simulink model "Scenario_17_v2"  (R2020b)
settings: Solver=ode1  StartTime=0.0  StopTime=10  FixedStep=Ts  MaxStep=Ts  MinStep=Ts/50  RelTol=1e-3
values from neighbouring files (symbols this model uses):
  c0 = c0_zeb    (= 6.57988e-09)    [Scenario_17_parameters_v2.m]    (also in Scenario_1_parameters_v2.m; Scenario_2_parameters_v2.m; Scenario_3_parameters_v2.m)
  c1 = c1_zeb    (= 9.15905e-09)    [Scenario_17_parameters_v2.m]    (also in Scenario_1_parameters_v2.m; Scenario_2_parameters_v2.m; Scenario_3_parameters_v2.m)
  fg = 50    [Scenario_17_parameters_v2.m]    (also in Scenario_1_parameters_v2.m; Scenario_2_parameters_v2.m; Scenario_3_parameters_v2.m)
  G11gen = 0.50    (= 0.5)    [Scenario_17_parameters_v2.m]
  G1gen = 0.4692    [Scenario_17_parameters_v2.m]    (also in Scenario_1_parameters_v2.m = 0.1; Scenario_2_parameters_v2.m = 0.298581; Scenario_3_parameters_v2.m = 0.65)
  G5gen = 0.75    [Scenario_17_parameters_v2.m]    (also in Scenario_1_parameters_v2.m = 0.8; Scenario_2_parameters_v2.m = 0.8; Scenario_3_parameters_v2.m = 0.705)
  G6gen = 0.90    (= 0.9)    [Scenario_17_parameters_v2.m]    (also in Scenario_1_parameters_v2.m; Scenario_2_parameters_v2.m = 0.81797; Scenario_3_parameters_v2.m = 0.45)
  G7gen = 0.20    (= 0.2)    [Scenario_17_parameters_v2.m]    (also in Scenario_1_parameters_v2.m = 0.5227; Scenario_2_parameters_v2.m = 0.5098; Scenario_3_parameters_v2.m = 0.4)
  G8gen = 0.58    [Scenario_17_parameters_v2.m]    (also in Scenario_3_parameters_v2.m = 0.65)
  G9gen = 0.8833    [Scenario_17_parameters_v2.m]    (also in Scenario_3_parameters_v2.m = 0.9)
  Iovc = 1.2    [Scenario_17_parameters_v2.m]    (also in Scenario_1_parameters_v2.m; Scenario_2_parameters_v2.m; Scenario_3_parameters_v2.m)
  l0 = l0_zeb    (= 0.00368)    [Scenario_17_parameters_v2.m]    (also in Scenario_1_parameters_v2.m; Scenario_2_parameters_v2.m; Scenario_3_parameters_v2.m)
  l1 = l1_zeb    (= 0.00128)    [Scenario_17_parameters_v2.m]    (also in Scenario_1_parameters_v2.m; Scenario_2_parameters_v2.m; Scenario_3_parameters_v2.m)
  L11dem = 0.02    [Scenario_17_parameters_v2.m]
  L12dem = 0.01    [Scenario_17_parameters_v2.m]    (also in Scenario_3_parameters_v2.m = 0.02)
  L1dem = 0.25    [Scenario_17_parameters_v2.m]    (also in Scenario_3_parameters_v2.m = 0.1)
  L3dem = 0.30    (= 0.3)    [Scenario_17_parameters_v2.m]    (also in Scenario_1_parameters_v2.m = 0.1; Scenario_2_parameters_v2.m = 0.1; Scenario_3_parameters_v2.m = 0.2)
  L5dem = 0.25    [Scenario_17_parameters_v2.m]    (also in Scenario_1_parameters_v2.m = 0.35; Scenario_2_parameters_v2.m = 0.35; Scenario_3_parameters_v2.m = 0.1)
  L9dem = 0.15    [Scenario_17_parameters_v2.m]    (also in Scenario_3_parameters_v2.m = 0.1)
  Pr = Sr*PF    (= 1600500000)    [Scenario_17_parameters_v2.m]    (also in Scenario_1_parameters_v2.m = 1472500000; Scenario_2_parameters_v2.m = 1805000000; Scenario_3_parameters_v2.m = 12740000000)
  Qr = sqrt(Sr^2 - Pr^2)    [Scenario_17_parameters_v2.m]    (also in Scenario_1_parameters_v2.m; Scenario_2_parameters_v2.m; Scenario_3_parameters_v2.m)
  r0 = r0_zeb    (= 0.39362)    [Scenario_17_parameters_v2.m]    (also in Scenario_1_parameters_v2.m; Scenario_2_parameters_v2.m; Scenario_3_parameters_v2.m)
  r1 = r1_zeb    (= 0.06862)    [Scenario_17_parameters_v2.m]    (also in Scenario_1_parameters_v2.m; Scenario_2_parameters_v2.m; Scenario_3_parameters_v2.m)
  Rtpu = Xtpu/40    (= 0.0025)    [Scenario_17_parameters_v2.m]    (also in Scenario_1_parameters_v2.m = 0.00375; Scenario_2_parameters_v2.m = 0.00375; Scenario_3_parameters_v2.m)
  S11non = 50e6    (= 50000000)    [Scenario_17_parameters_v2.m]
  S1non = 700e6    (= 700000000)    [Scenario_17_parameters_v2.m]    (also in Scenario_1_parameters_v2.m = 400000000; Scenario_2_parameters_v2.m = 400000000; Scenario_3_parameters_v2.m = 1000000000)
  S5non = 400e6    (= 400000000)    [Scenario_17_parameters_v2.m]    (also in Scenario_1_parameters_v2.m = 500000000; Scenario_2_parameters_v2.m = 500000000; Scenario_3_parameters_v2.m = 2000000000)
  S6non = 150e6    (= 150000000)    [Scenario_17_parameters_v2.m]    (also in Scenario_1_parameters_v2.m = 400000000; Scenario_2_parameters_v2.m = 400000000; Scenario_3_parameters_v2.m = 3000000000)
  S7non = 1500e6    (= 1500000000)    [Scenario_17_parameters_v2.m]    (also in Scenario_1_parameters_v2.m = 200000000; Scenario_2_parameters_v2.m = 200000000; Scenario_3_parameters_v2.m = 4000000000)
  S8non = 600e6    (= 600000000)    [Scenario_17_parameters_v2.m]    (also in Scenario_3_parameters_v2.m = 2000000000)
  S9non = 200e6    (= 200000000)    [Scenario_17_parameters_v2.m]    (also in Scenario_3_parameters_v2.m = 1500000000)
  tonvsc = 0    [Scenario_17_parameters_v2.m]    (also in Scenario_1_parameters_v2.m; Scenario_2_parameters_v2.m; Scenario_3_parameters_v2.m = 0.0001)
  Ts = 50e-6    (= 5e-05)    [Scenario_17_parameters_v2.m]    (also in Scenario_1_parameters_v2.m = 0.0002; Scenario_2_parameters_v2.m = 2e-05; Scenario_3_parameters_v2.m = 0.0001)
  Vhv = 220e3    (= 220000)    [Scenario_17_parameters_v2.m]    (also in Scenario_1_parameters_v2.m; Scenario_2_parameters_v2.m; Scenario_3_parameters_v2.m)
  Vmv = 22e3    (= 22000)    [Scenario_17_parameters_v2.m]    (also in Scenario_1_parameters_v2.m; Scenario_2_parameters_v2.m; Scenario_3_parameters_v2.m)
  w_pll = 2*pi*80    (= 502.654824574)    [Scenario_17_parameters_v2.m]    (also in Scenario_1_parameters_v2.m; Scenario_2_parameters_v2.m; Scenario_3_parameters_v2.m)
  wc1 = wsw1/10    (= 848.230016469)    [Scenario_17_parameters_v2.m]    (also in Scenario_1_parameters_v2.m; Scenario_2_parameters_v2.m; Scenario_3_parameters_v2.m)
  wdc1 = wc1/10    (= 84.8230016469)    [Scenario_17_parameters_v2.m]    (also in Scenario_1_parameters_v2.m; Scenario_2_parameters_v2.m; Scenario_3_parameters_v2.m)
  wpq1 = wc1/10    (= 84.8230016469)    [Scenario_17_parameters_v2.m]    (also in Scenario_1_parameters_v2.m; Scenario_2_parameters_v2.m; Scenario_3_parameters_v2.m)
  wsw1 = ksw1*2*pi*fg    (= 8482.30016469)    [Scenario_17_parameters_v2.m]    (also in Scenario_1_parameters_v2.m; Scenario_2_parameters_v2.m; Scenario_3_parameters_v2.m)
  Xtpu = 0.10    (= 0.1)    [Scenario_17_parameters_v2.m]    (also in Scenario_1_parameters_v2.m = 0.15; Scenario_2_parameters_v2.m = 0.15; Scenario_3_parameters_v2.m)
undefined symbols (not defined in the file or in its folder): D11, Delta, Newton, Raphson
libraries: powerlib x349, simulink_extras x215, powerlib_meascontrol x165, pid_lib x81, simulink x48, eeTransforms x42, spsFirstOrderFilterLib x28, eePwmGeneratorTwoLevel x7
(part 4 of 31)

== system Scenario_17_v2/HVDC 1 ==
  note: Converter controlling DC voltage
  note: DC Link dynamics
  note: avoid division by zero
  note: avoid division by zero
  Bus Selector1 : BusSelector  OutputSignals=Pabc,Qabc,f
  Bus Selector2 : BusSelector  OutputSignals=Pabc,Qabc,f
  Constant : Constant  Value=-S7non*G7gen
  Constant1 : Constant  Value=0
  Constant2 : Constant  Value=100e6
  DC-link : Subsystem  mask{C1=3100e-6/2, C2=3100e-6/2, R=4, L=100e-3, Vdc0=2*Vhv*sqrt(2)/sqrt(3), Pdc0=S7non*G7gen}
      mask prompts: C1 "Terminal 1 capacitance (F)"; C2 "Termina 2 capacitance (F)"; R "Link series resistance (Ohm)"; L "Link series inductance (H)"; Vdc0 "Link Initial voltage (V)"; Pdc0 "Initial power flowing from 1 to 2"
      mask init:
      | idc0 = Pdc0/Vdc0;
      | v2dc0 = Vdc0; % Initial voltage of terminal 2
      | v1dc0 = Vdc0 + idc0*R; % Initial voltage of terminal 1
      mask Display:
      | disp('back-to-back\n')
      | disp('\nDC link')
  Divide : Product  Inputs=*/
  Divide1 : Product  Inputs=*/
  Gain1 : Gain  Gain=-1
  Gain2 : Gain  Gain=-1
  Saturation : Saturate  UpperLimit=5*Vhv  LowerLimit=0.01*Vhv
  Saturation1 : Saturate  UpperLimit=5*Vhv  LowerLimit=0.01*Vhv
  Unit Delay : UnitDelay  SampleTime=-1  HasFrameUpgradeWarning=on
  Unit Delay1 : UnitDelay  SampleTime=-1  HasFrameUpgradeWarning=on
  VSC1 : Subsystem  mask{vscmod=EMT Average, fg=fg, Vhv=Vhv, Vmv=Vhv, Pconv=S7non, Rtpu=Rtpu, Xtpu=Xtpu, qmode=Active power, dmode=Reactive power, wsw=wsw1, wn_pll=w_pll, wc=wc1, wpq=wpq1, wdc=wdc1, koc=Iovc, Cdc=3100e-6, tfilt=1*(1/wsw1), negseq_en=off, fdroop_en=off, Vacdroop_en=off, LVRT_en=off, Kfdroop=0.05, fdroop_per=10, Kvdroop=0.1, Vacdroop_per=10, Vlvrt0=0.9, Vlvrt_min=0.5, Qmax_lvrt=0.9, V0pu=1, theta0=0, P0=-S7non*G7gen, Q0=0}
      mask prompts: vscmod "VSC Model"; fg "AC grid frequency (Hz)"; Vhv "Grid-side voltage (V)(LL-rms)"; Vmv "Converter-side voltage (V)(LL-rms)"; Pconv "Converter nominal power (VA)"; Rtpu "Resistance seen by the converter (p.u)"; Xtpu "Reactance seen by the converter (p.u)"; qmode "q-axis control mode"; dmode "d-axis control mode"; wsw "Switching frequency (rad/s)"; wn_pll "PLL filter natural frequency"; wc "Current-control bandwidth (rad/s)"; wpq "PQ control bandwidth (rad/s)"; wdc "DC Voltage control bandwidth(rad/s)"; koc "Overcurrent factor (p.u)"; Cdc "DC-side total capacitance (F)"; tfilt "Vabc filter time constant (s)"; negseq_en "Enable negative sequence control"; fdroop_en "Enable frequency droop"; Vacdroop_en "Enable AC voltage droop"; LVRT_en "Enable LVRT"; Kfdroop "Frequency droop (p.u)"; fdroop_per "Percentage of converter power to contribute with droop (%)"; Kvdroop "Voltage droop (p.u)"; Vacdroop_per "Percentage of converter power to contribute with droop (%)"; Vlvrt0 "initial voltage (p.u)"; Vlvrt_min "minimum voltage (p.u)"; Qmax_lvrt "max power injected at min voltage (p.u)"; V0pu "Initial terminal voltage magnitude (pu)"; theta0 "Initial terminal voltage angle (deg)"; P0 "Initial active power (W)"; Q0 "Initial reactive power (VAr)"
      mask init: same as Scenario_17_v2/G11new/VSC v2
      mask TypeOptions vscmod: EMT Switching | EMT Average | Phasor Quasi-EMT | Phasor I-1st | Phasor I-ref | Phasor PQ-1st
      mask Callback vscmod:
      | % Control parameter visiblity
      | 
      | % Get the value of the Enable Bias checkbox
      | % unchecked = 'off'
      | % checked = 'on'
      | 
      | maskObj = Simulink.Mask.get(gcb);
      | 
      | wn_pll = 'on';
      | wsw = 'on';
      | DC_en = 'off';
      | 
      | vscmod = get_param(gcb,'vscmod');
      |     if strcmp(vscmod,'EMT Switching')
      |       wn_pll = 'on';
      |       wsw = 'on';
      |       tfilt = 'on';
      |     elseif strcmp(vscmod,'EMT Average')
      |         wn_pll = 'on';
      |         wsw = 'off';
      |         tfilt = 'off';
      |     elseif strcmp(vscmod,'Phasor Quasi-EMT')
      |         wn_pll = 'off';
      |         wsw = 'off';
      |         tfilt = 'off';
      |     elseif strcmp(vscmod,'Phasor I-1st')
      |         wn_pll = 'off';
      |         wsw = 'off';
      |         tfilt = 'off';
      |     elseif strcmp(vscmod,'Phasor I-ref')
      |         wn_pll = 'off';
      |         wsw = 'off';
      |         tfilt = 'off';
      |     elseif strcmp(vscmod,'Phasor PQ-1st')
      |         wn_pll = 'off';
      |         wsw = 'off';
      |         tfilt = 'off';
      |     end
      | 
      | fdroop_en = get_param(gcb,'fdroop_en');
      | Vacdroop_en = get_param(gcb,'Vacdroop_en');
      | LVRT_en = get_param(gcb,'LVRT_en');
      | negseq_en = get_param(gcb,'negseq_en');
      | qmode_str = get_param(gcb,'qmode');
      | 
      | 
      | if strcmp(qmode_str,'DC voltage')
      |     DC_en = 'on';
      | else
      |     DC_en = 'off';
      | end
      | 
      | % Set the 'MaskVisibilities' property for each parameters
      |     set_param(gcb,'MaskVisibilities',{'on','on','on','on','on','on','on','on','on',wsw,wn_pll,'on','on','on','on',DC_en,tfilt,'on','on','on','on',fdroop_en,fdroop_en,Vacdroop_en,Vacdroop_en,'on','on','on','on','on','on','on'});
      | 
      | % Make LVRT area visible when it is enabled
      | if strcmp(LVRT_en,'on')
      |   maskObj.getDialogControl('Container_LVRT').Visible = 'on';
      | else
      |     maskObj.getDialogControl('Container_LVRT').Visible = 'off';
      | end
      | 
      | % Note that the value of the bias is not handled here.
      | % See the Initialization tab
      mask TypeOptions qmode: Active power | DC voltage
      mask Callback qmode:
      | % Control parameter visiblity
      | 
      | % Get the value of the Enable Bias checkbox
      | % unchecked = 'off'
      | % checked = 'on'
      | 
      | maskObj = Simulink.Mask.get(gcb);
      | 
      | wn_pll = 'on';
      | wsw = 'on';
      | DC_en = 'off';
      | 
      | vscmod = get_param(gcb,'vscmod');
      |     if strcmp(vscmod,'EMT Switching')
      |       wn_pll = 'on';
      |       wsw = 'on';
      |       tfilt = 'on';
      |     elseif strcmp(vscmod,'EMT Average')
      |         wn_pll = 'on';
      |         wsw = 'off';
      |         tfilt = 'off';
      |     elseif strcmp(vscmod,'Phasor Quasi-EMT')
      |         wn_pll = 'off';
      |         wsw = 'off';
      |         tfilt = 'off';
      |     elseif strcmp(vscmod,'Phasor I-1st')
      |         wn_pll = 'off';
      |         wsw = 'off';
      |         tfilt = 'off';
      |     elseif strcmp(vscmod,'Phasor I-ref')
      |         wn_pll = 'off';
      |         wsw = 'off';
      |         tfilt = 'off';
      |     elseif strcmp(vscmod,'Phasor PQ-1st')
      |         wn_pll = 'off';
      |         wsw = 'off';
      |         tfilt = 'off';
      |     end
      | 
      | fdroop_en = get_param(gcb,'fdroop_en');
      | Vacdroop_en = get_param(gcb,'Vacdroop_en');
      | LVRT_en = get_param(gcb,'LVRT_en');
      | negseq_en = get_param(gcb,'negseq_en');
      | qmode_str = get_param(gcb,'qmode');
      | 
      | 
      | if strcmp(qmode_str,'DC voltage')
      |     DC_en = 'on';
      | else
      |     DC_en = 'off';
      | end
      | 
      | % Set the 'MaskVisibilities' property for each parameters
      |     set_param(gcb,'MaskVisibilities',{'on','on','on','on','on','on','on','on','on',wsw,wn_pll,'on','on','on','on',DC_en,tfilt,'on','on','on','on',fdroop_en,fdroop_en,Vacdroop_en,Vacdroop_en,'on','on','on','on','on','on','on'});
      | 
      | % Make LVRT area visible when it is enabled
      | if strcmp(LVRT_en,'on')
      |   maskObj.getDialogControl('Container_LVRT').Visible = 'on';
      | else
      |     maskObj.getDialogControl('Container_LVRT').Visible = 'off';
      | end
      | 
      | % Note that the value of the bias is not handled here.
      | % See the Initialization tab
      mask TypeOptions dmode: Reactive power | AC voltage
      mask Callback fdroop_en:
      | % Control parameter visiblity
      | 
      | % Get the value of the Enable Bias checkbox
      | % unchecked = 'off'
      | % checked = 'on'
      | 
      | maskObj = Simulink.Mask.get(gcb);
      | 
      | wn_pll = 'on';
      | wsw = 'on';
      | DC_en = 'off';
      | 
      | vscmod = get_param(gcb,'vscmod');
      |     if strcmp(vscmod,'EMT Switching')
      |       wn_pll = 'on';
      |       wsw = 'on';
      |       tfilt = 'on';
      |     elseif strcmp(vscmod,'EMT Average')
      |         wn_pll = 'on';
      |         wsw = 'off';
      |         tfilt = 'off';
      |     elseif strcmp(vscmod,'Phasor Quasi-EMT')
      |         wn_pll = 'off';
      |         wsw = 'off';
      |         tfilt = 'off';
      |     elseif strcmp(vscmod,'Phasor I-1st')
      |         wn_pll = 'off';
      |         wsw = 'off';
      |         tfilt = 'off';
      |     elseif strcmp(vscmod,'Phasor I-ref')
      |         wn_pll = 'off';
      |         wsw = 'off';
      |         tfilt = 'off';
      |     elseif strcmp(vscmod,'Phasor PQ-1st')
      |         wn_pll = 'off';
      |         wsw = 'off';
      |         tfilt = 'off';
      |     end
      | 
      | fdroop_en = get_param(gcb,'fdroop_en');
      | Vacdroop_en = get_param(gcb,'Vacdroop_en');
      | LVRT_en = get_param(gcb,'LVRT_en');
      | negseq_en = get_param(gcb,'negseq_en');
      | qmode_str = get_param(gcb,'qmode');
      | 
      | 
      | if strcmp(qmode_str,'DC voltage')
      |     DC_en = 'on';
      | else
      |     DC_en = 'off';
      | end
      | 
      | % Set the 'MaskVisibilities' property for each parameters
      |     set_param(gcb,'MaskVisibilities',{'on','on','on','on','on','on','on','on','on',wsw,wn_pll,'on','on','on','on',DC_en,tfilt,'on','on','on','on',fdroop_en,fdroop_en,Vacdroop_en,Vacdroop_en,'on','on','on','on','on','on','on'});
      | 
      | % Make LVRT area visible when it is enabled
      | if strcmp(LVRT_en,'on')
      |   maskObj.getDialogControl('Container_LVRT').Visible = 'on';
      | else
      |     maskObj.getDialogControl('Container_LVRT').Visible = 'off';
      | end
      | 
      | % Note that the value of the bias is not handled here.
      | % See the Initialization tab
      mask Callback Vacdroop_en:
      | % Control parameter visiblity
      | 
      | % Get the value of the Enable Bias checkbox
      | % unchecked = 'off'
      | % checked = 'on'
      | 
      | maskObj = Simulink.Mask.get(gcb);
      | 
      | wn_pll = 'on';
      | wsw = 'on';
      | DC_en = 'off';
      | 
      | vscmod = get_param(gcb,'vscmod');
      |     if strcmp(vscmod,'EMT Switching')
      |       wn_pll = 'on';
      |       wsw = 'on';
      |       tfilt = 'on';
      |     elseif strcmp(vscmod,'EMT Average')
      |         wn_pll = 'on';
      |         wsw = 'off';
      |         tfilt = 'off';
      |     elseif strcmp(vscmod,'Phasor Quasi-EMT')
      |         wn_pll = 'off';
      |         wsw = 'off';
      |         tfilt = 'off';
      |     elseif strcmp(vscmod,'Phasor I-1st')
      |         wn_pll = 'off';
      |         wsw = 'off';
      |         tfilt = 'off';
      |     elseif strcmp(vscmod,'Phasor I-ref')
      |         wn_pll = 'off';
      |         wsw = 'off';
      |         tfilt = 'off';
      |     elseif strcmp(vscmod,'Phasor PQ-1st')
      |         wn_pll = 'off';
      |         wsw = 'off';
      |         tfilt = 'off';
      |     end
      | 
      | fdroop_en = get_param(gcb,'fdroop_en');
      | Vacdroop_en = get_param(gcb,'Vacdroop_en');
      | LVRT_en = get_param(gcb,'LVRT_en');
      | negseq_en = get_param(gcb,'negseq_en');
      | qmode_str = get_param(gcb,'qmode');
      | 
      | 
      | if strcmp(qmode_str,'DC voltage')
      |     DC_en = 'on';
      | else
      |     DC_en = 'off';
      | end
      | 
      | % Set the 'MaskVisibilities' property for each parameters
      |     set_param(gcb,'MaskVisibilities',{'on','on','on','on','on','on','on','on','on',wsw,wn_pll,'on','on','on','on',DC_en,tfilt,'on','on','on','on',fdroop_en,fdroop_en,Vacdroop_en,Vacdroop_en,'on','on','on','on','on','on','on'});
      | 
      | % Make LVRT area visible when it is enabled
      | if strcmp(LVRT_en,'on')
      |   maskObj.getDialogControl('Container_LVRT').Visible = 'on';
      | else
      |     maskObj.getDialogControl('Container_LVRT').Visible = 'off';
      | end
      | 
      | % Note that the value of the bias is not handled here.
      | % See the Initialization tab
      mask Callback LVRT_en:
      | % Control parameter visiblity
      | 
      | % Get the value of the Enable Bias checkbox
      | % unchecked = 'off'
      | % checked = 'on'
      | 
      | maskObj = Simulink.Mask.get(gcb);
      | 
      | wn_pll = 'on';
      | wsw = 'on';
      | DC_en = 'off';
      | 
      | vscmod = get_param(gcb,'vscmod');
      |     if strcmp(vscmod,'EMT Switching')
      |       wn_pll = 'on';
      |       wsw = 'on';
      |       tfilt = 'on';
      |     elseif strcmp(vscmod,'EMT Average')
      |         wn_pll = 'on';
      |         wsw = 'off';
      |         tfilt = 'off';
      |     elseif strcmp(vscmod,'Phasor Quasi-EMT')
      |         wn_pll = 'off';
      |         wsw = 'off';
      |         tfilt = 'off';
      |     elseif strcmp(vscmod,'Phasor I-1st')
      |         wn_pll = 'off';
      |         wsw = 'off';
      |         tfilt = 'off';
      |     elseif strcmp(vscmod,'Phasor I-ref')
      |         wn_pll = 'off';
      |         wsw = 'off';
      |         tfilt = 'off';
      |     elseif strcmp(vscmod,'Phasor PQ-1st')
      |         wn_pll = 'off';
      |         wsw = 'off';
      |         tfilt = 'off';
      |     end
      | 
      | fdroop_en = get_param(gcb,'fdroop_en');
      | Vacdroop_en = get_param(gcb,'Vacdroop_en');
      | LVRT_en = get_param(gcb,'LVRT_en');
      | negseq_en = get_param(gcb,'negseq_en');
      | qmode_str = get_param(gcb,'qmode');
      | 
      | 
      | if strcmp(qmode_str,'DC voltage')
      |     DC_en = 'on';
      | else
      |     DC_en = 'off';
      | end
      | 
      | % Set the 'MaskVisibilities' property for each parameters
      |     set_param(gcb,'MaskVisibilities',{'on','on','on','on','on','on','on','on','on',wsw,wn_pll,'on','on','on','on',DC_en,tfilt,'on','on','on','on',fdroop_en,fdroop_en,Vacdroop_en,Vacdroop_en,'on','on','on','on','on','on','on'});
      | 
      | % Make LVRT area visible when it is enabled
      | if strcmp(LVRT_en,'on')
      |   maskObj.getDialogControl('Container_LVRT').Visible = 'on';
      | else
      |     maskObj.getDialogControl('Container_LVRT').Visible = 'off';
      | end
      | 
      | % Note that the value of the bias is not handled here.
      | % See the Initialization tab
      mask DialogControl DescTextVar Prompt: -------------------------------------Three-phase VSC model---------------------------------------
      mask DialogControl Tab1 Prompt: Electrical parameters
      mask DialogControl Tab2 Prompt: Control parameters
      mask DialogControl Tab3 Prompt: Other parameters
      mask DialogControl Container_LVRT Prompt: LVRT
      mask DialogControl Tab4 Prompt: Power flow
      mask Display:
      | choice = get_param(gcb,'vscmod');
      | if strcmp(choice,'Phasor Quasi-EMT')
      |     disp('VSC\n\n')
      |     disp('\n\nPhasor\n\n')
      |     disp('\n\nQuasi-EMT')
      | elseif strcmp(choice,'EMT Average')
      |     disp('VSC\n')
      |     disp('\nEMT AVG')
      | elseif strcmp(choice,'EMT Switching')
      |     disp('VSC\n')
      |     disp('\nEMT SW')
      | elseif strcmp(choice,'Phasor I-1st')
      |     disp('VSC\n\n')
      |     disp('\n\nPhasor\n\n')
      |     disp('\n\nI 1st')
      | elseif strcmp(choice,'Phasor I-ref')
      |     disp('VSC\n\n')
      |     disp('\n\nPhasor\n\n')
      |     disp('\n\nI ref')
      | elseif strcmp(choice,'Phasor PQ-1st')
      |     disp('VSC\n\n')
      |     disp('\n\nPhasor\n\n')
      |     disp('\n\nPQ 1st')
      | end
  VSC2 : Subsystem  mask{vscmod=EMT Average, fg=fg, Vhv=Vhv, Vmv=Vhv, Pconv=S7non, Rtpu=Rtpu, Xtpu=Xtpu, qmode=DC voltage, dmode=Reactive power, wsw=wsw1, wn_pll=w_pll, wc=wc1, wpq=wpq1, wdc=wdc1, koc=Iovc, Cdc=3100e-6, tfilt=1*(1/wsw1), negseq_en=off, fdroop_en=off, Vacdroop_en=off, LVRT_en=off, Kfdroop=0.05, fdroop_per=10, Kvdroop=0.1, Vacdroop_per=10, Vlvrt0=0.9, Vlvrt_min=0.5, Qmax_lvrt=0.9, V0pu=1.0433, theta0=-29.85, P0=S7non*G7gen, Q0=100e6}
      mask prompts: vscmod "VSC Model"; fg "AC grid frequency (Hz)"; Vhv "Grid-side voltage (V)(LL-rms)"; Vmv "Converter-side voltage (V)(LL-rms)"; Pconv "Converter nominal power (VA)"; Rtpu "Resistance seen by the converter (p.u)"; Xtpu "Reactance seen by the converter (p.u)"; qmode "q-axis control mode"; dmode "d-axis control mode"; wsw "Switching frequency (rad/s)"; wn_pll "PLL filter natural frequency"; wc "Current-control bandwidth (rad/s)"; wpq "PQ control bandwidth (rad/s)"; wdc "DC Voltage control bandwidth(rad/s)"; koc "Overcurrent factor (p.u)"; Cdc "DC-side total capacitance (F)"; tfilt "Vabc filter time constant (s)"; negseq_en "Enable negative sequence control"; fdroop_en "Enable frequency droop"; Vacdroop_en "Enable AC voltage droop"; LVRT_en "Enable LVRT"; Kfdroop "Frequency droop (p.u)"; fdroop_per "Percentage of converter power to contribute with droop (%)"; Kvdroop "Voltage droop (p.u)"; Vacdroop_per "Percentage of converter power to contribute with droop (%)"; Vlvrt0 "initial voltage (p.u)"; Vlvrt_min "minimum voltage (p.u)"; Qmax_lvrt "max power injected at min voltage (p.u)"; V0pu "Initial terminal voltage magnitude (pu)"; theta0 "Initial terminal voltage angle (deg)"; P0 "Initial active power (W)"; Q0 "Initial reactive power (VAr)"
      mask init: same as Scenario_17_v2/G11new/VSC v2
      mask TypeOptions vscmod: EMT Switching | EMT Average | Phasor Quasi-EMT | Phasor I-1st | Phasor I-ref | Phasor PQ-1st
      mask Callback vscmod:
      | % Control parameter visiblity
      | 
      | % Get the value of the Enable Bias checkbox
      | % unchecked = 'off'
      | % checked = 'on'
      | 
      | maskObj = Simulink.Mask.get(gcb);
      | 
      | wn_pll = 'on';
      | wsw = 'on';
      | DC_en = 'off';
      | 
      | vscmod = get_param(gcb,'vscmod');
      |     if strcmp(vscmod,'EMT Switching')
      |       wn_pll = 'on';
      |       wsw = 'on';
      |       tfilt = 'on';
      |     elseif strcmp(vscmod,'EMT Average')
      |         wn_pll = 'on';
      |         wsw = 'off';
      |         tfilt = 'off';
      |     elseif strcmp(vscmod,'Phasor Quasi-EMT')
      |         wn_pll = 'off';
      |         wsw = 'off';
      |         tfilt = 'off';
      |     elseif strcmp(vscmod,'Phasor I-1st')
      |         wn_pll = 'off';
      |         wsw = 'off';
      |         tfilt = 'off';
      |     elseif strcmp(vscmod,'Phasor I-ref')
      |         wn_pll = 'off';
      |         wsw = 'off';
      |         tfilt = 'off';
      |     elseif strcmp(vscmod,'Phasor PQ-1st')
      |         wn_pll = 'off';
      |         wsw = 'off';
      |         tfilt = 'off';
      |     end
      | 
      | fdroop_en = get_param(gcb,'fdroop_en');
      | Vacdroop_en = get_param(gcb,'Vacdroop_en');
      | LVRT_en = get_param(gcb,'LVRT_en');
      | negseq_en = get_param(gcb,'negseq_en');
      | qmode_str = get_param(gcb,'qmode');
      | 
      | 
      | if strcmp(qmode_str,'DC voltage')
      |     DC_en = 'on';
      | else
      |     DC_en = 'off';
      | end
      | 
      | % Set the 'MaskVisibilities' property for each parameters
      |     set_param(gcb,'MaskVisibilities',{'on','on','on','on','on','on','on','on','on',wsw,wn_pll,'on','on','on','on',DC_en,tfilt,'on','on','on','on',fdroop_en,fdroop_en,Vacdroop_en,Vacdroop_en,'on','on','on','on','on','on','on'});
      | 
      | % Make LVRT area visible when it is enabled
      | if strcmp(LVRT_en,'on')
      |   maskObj.getDialogControl('Container_LVRT').Visible = 'on';
      | else
      |     maskObj.getDialogControl('Container_LVRT').Visible = 'off';
      | end
      | 
      | % Note that the value of the bias is not handled here.
      | % See the Initialization tab
      mask TypeOptions qmode: Active power | DC voltage
      mask Callback qmode:
      | % Control parameter visiblity
      | 
      | % Get the value of the Enable Bias checkbox
      | % unchecked = 'off'
      | % checked = 'on'
      | 
      | maskObj = Simulink.Mask.get(gcb);
      | 
      | wn_pll = 'on';
      | wsw = 'on';
      | DC_en = 'off';
      | 
      | vscmod = get_param(gcb,'vscmod');
      |     if strcmp(vscmod,'EMT Switching')
      |       wn_pll = 'on';
      |       wsw = 'on';
      |       tfilt = 'on';
      |     elseif strcmp(vscmod,'EMT Average')
      |         wn_pll = 'on';
      |         wsw = 'off';
      |         tfilt = 'off';
      |     elseif strcmp(vscmod,'Phasor Quasi-EMT')
      |         wn_pll = 'off';
      |         wsw = 'off';
      |         tfilt = 'off';
      |     elseif strcmp(vscmod,'Phasor I-1st')
      |         wn_pll = 'off';
      |         wsw = 'off';
      |         tfilt = 'off';
      |     elseif strcmp(vscmod,'Phasor I-ref')
      |         wn_pll = 'off';
      |         wsw = 'off';
      |         tfilt = 'off';
      |     elseif strcmp(vscmod,'Phasor PQ-1st')
      |         wn_pll = 'off';
      |         wsw = 'off';
      |         tfilt = 'off';
      |     end
      | 
      | fdroop_en = get_param(gcb,'fdroop_en');
      | Vacdroop_en = get_param(gcb,'Vacdroop_en');
      | LVRT_en = get_param(gcb,'LVRT_en');
      | negseq_en = get_param(gcb,'negseq_en');
      | qmode_str = get_param(gcb,'qmode');
      | 
      | 
      | if strcmp(qmode_str,'DC voltage')
      |     DC_en = 'on';
      | else
      |     DC_en = 'off';
      | end
      | 
      | % Set the 'MaskVisibilities' property for each parameters
      |     set_param(gcb,'MaskVisibilities',{'on','on','on','on','on','on','on','on','on',wsw,wn_pll,'on','on','on','on',DC_en,tfilt,'on','on','on','on',fdroop_en,fdroop_en,Vacdroop_en,Vacdroop_en,'on','on','on','on','on','on','on'});
      | 
      | % Make LVRT area visible when it is enabled
      | if strcmp(LVRT_en,'on')
      |   maskObj.getDialogControl('Container_LVRT').Visible = 'on';
      | else
      |     maskObj.getDialogControl('Container_LVRT').Visible = 'off';
      | end
      | 
      | % Note that the value of the bias is not handled here.
      | % See the Initialization tab
      mask TypeOptions dmode: Reactive power | AC voltage
      mask Callback fdroop_en:
      | % Control parameter visiblity
      | 
      | % Get the value of the Enable Bias checkbox
      | % unchecked = 'off'
      | % checked = 'on'
      | 
      | maskObj = Simulink.Mask.get(gcb);
      | 
      | wn_pll = 'on';
      | wsw = 'on';
      | DC_en = 'off';
      | 
      | vscmod = get_param(gcb,'vscmod');
      |     if strcmp(vscmod,'EMT Switching')
      |       wn_pll = 'on';
      |       wsw = 'on';
      |       tfilt = 'on';
      |     elseif strcmp(vscmod,'EMT Average')
      |         wn_pll = 'on';
      |         wsw = 'off';
      |         tfilt = 'off';
      |     elseif strcmp(vscmod,'Phasor Quasi-EMT')
      |         wn_pll = 'off';
      |         wsw = 'off';
      |         tfilt = 'off';
      |     elseif strcmp(vscmod,'Phasor I-1st')
      |         wn_pll = 'off';
      |         wsw = 'off';
      |         tfilt = 'off';
      |     elseif strcmp(vscmod,'Phasor I-ref')
      |         wn_pll = 'off';
      |         wsw = 'off';
      |         tfilt = 'off';
      |     elseif strcmp(vscmod,'Phasor PQ-1st')
      |         wn_pll = 'off';
      |         wsw = 'off';
      |         tfilt = 'off';
      |     end
      | 
      | fdroop_en = get_param(gcb,'fdroop_en');
      | Vacdroop_en = get_param(gcb,'Vacdroop_en');
      | LVRT_en = get_param(gcb,'LVRT_en');
      | negseq_en = get_param(gcb,'negseq_en');
      | qmode_str = get_param(gcb,'qmode');
      | 
      | 
      | if strcmp(qmode_str,'DC voltage')
      |     DC_en = 'on';
      | else
      |     DC_en = 'off';
      | end
      | 
      | % Set the 'MaskVisibilities' property for each parameters
      |     set_param(gcb,'MaskVisibilities',{'on','on','on','on','on','on','on','on','on',wsw,wn_pll,'on','on','on','on',DC_en,tfilt,'on','on','on','on',fdroop_en,fdroop_en,Vacdroop_en,Vacdroop_en,'on','on','on','on','on','on','on'});
      | 
      | % Make LVRT area visible when it is enabled
      | if strcmp(LVRT_en,'on')
      |   maskObj.getDialogControl('Container_LVRT').Visible = 'on';
      | else
      |     maskObj.getDialogControl('Container_LVRT').Visible = 'off';
      | end
      | 
      | % Note that the value of the bias is not handled here.
      | % See the Initialization tab
      mask Callback Vacdroop_en:
      | % Control parameter visiblity
      | 
      | % Get the value of the Enable Bias checkbox
      | % unchecked = 'off'
      | % checked = 'on'
      | 
      | maskObj = Simulink.Mask.get(gcb);
      | 
      | wn_pll = 'on';
      | wsw = 'on';
      | DC_en = 'off';
      | 
      | vscmod = get_param(gcb,'vscmod');
      |     if strcmp(vscmod,'EMT Switching')
      |       wn_pll = 'on';
      |       wsw = 'on';
      |       tfilt = 'on';
      |     elseif strcmp(vscmod,'EMT Average')
      |         wn_pll = 'on';
      |         wsw = 'off';
      |         tfilt = 'off';
      |     elseif strcmp(vscmod,'Phasor Quasi-EMT')
      |         wn_pll = 'off';
      |         wsw = 'off';
      |         tfilt = 'off';
      |     elseif strcmp(vscmod,'Phasor I-1st')
      |         wn_pll = 'off';
      |         wsw = 'off';
      |         tfilt = 'off';
      |     elseif strcmp(vscmod,'Phasor I-ref')
      |         wn_pll = 'off';
      |         wsw = 'off';
      |         tfilt = 'off';
      |     elseif strcmp(vscmod,'Phasor PQ-1st')
      |         wn_pll = 'off';
      |         wsw = 'off';
      |         tfilt = 'off';
      |     end
      | 
      | fdroop_en = get_param(gcb,'fdroop_en');
      | Vacdroop_en = get_param(gcb,'Vacdroop_en');
      | LVRT_en = get_param(gcb,'LVRT_en');
      | negseq_en = get_param(gcb,'negseq_en');
      | qmode_str = get_param(gcb,'qmode');
      | 
      | 
      | if strcmp(qmode_str,'DC voltage')
      |     DC_en = 'on';
      | else
      |     DC_en = 'off';
      | end
      | 
      | % Set the 'MaskVisibilities' property for each parameters
      |     set_param(gcb,'MaskVisibilities',{'on','on','on','on','on','on','on','on','on',wsw,wn_pll,'on','on','on','on',DC_en,tfilt,'on','on','on','on',fdroop_en,fdroop_en,Vacdroop_en,Vacdroop_en,'on','on','on','on','on','on','on'});
      | 
      | % Make LVRT area visible when it is enabled
      | if strcmp(LVRT_en,'on')
      |   maskObj.getDialogControl('Container_LVRT').Visible = 'on';
      | else
      |     maskObj.getDialogControl('Container_LVRT').Visible = 'off';
      | end
      | 
      | % Note that the value of the bias is not handled here.
      | % See the Initialization tab
      mask Callback LVRT_en:
      | % Control parameter visiblity
      | 
      | % Get the value of the Enable Bias checkbox
      | % unchecked = 'off'
      | % checked = 'on'
      | 
      | maskObj = Simulink.Mask.get(gcb);
      | 
      | wn_pll = 'on';
      | wsw = 'on';
      | DC_en = 'off';
      | 
      | vscmod = get_param(gcb,'vscmod');
      |     if strcmp(vscmod,'EMT Switching')
      |       wn_pll = 'on';
      |       wsw = 'on';
      |       tfilt = 'on';
      |     elseif strcmp(vscmod,'EMT Average')
      |         wn_pll = 'on';
      |         wsw = 'off';
      |         tfilt = 'off';
      |     elseif strcmp(vscmod,'Phasor Quasi-EMT')
      |         wn_pll = 'off';
      |         wsw = 'off';
      |         tfilt = 'off';
      |     elseif strcmp(vscmod,'Phasor I-1st')
      |         wn_pll = 'off';
      |         wsw = 'off';
      |         tfilt = 'off';
      |     elseif strcmp(vscmod,'Phasor I-ref')
      |         wn_pll = 'off';
      |         wsw = 'off';
      |         tfilt = 'off';
      |     elseif strcmp(vscmod,'Phasor PQ-1st')
      |         wn_pll = 'off';
      |         wsw = 'off';
      |         tfilt = 'off';
      |     end
      | 
      | fdroop_en = get_param(gcb,'fdroop_en');
      | Vacdroop_en = get_param(gcb,'Vacdroop_en');
      | LVRT_en = get_param(gcb,'LVRT_en');
      | negseq_en = get_param(gcb,'negseq_en');
      | qmode_str = get_param(gcb,'qmode');
      | 
      | 
      | if strcmp(qmode_str,'DC voltage')
      |     DC_en = 'on';
      | else
      |     DC_en = 'off';
      | end
      | 
      | % Set the 'MaskVisibilities' property for each parameters
      |     set_param(gcb,'MaskVisibilities',{'on','on','on','on','on','on','on','on','on',wsw,wn_pll,'on','on','on','on',DC_en,tfilt,'on','on','on','on',fdroop_en,fdroop_en,Vacdroop_en,Vacdroop_en,'on','on','on','on','on','on','on'});
      | 
      | % Make LVRT area visible when it is enabled
      | if strcmp(LVRT_en,'on')
      |   maskObj.getDialogControl('Container_LVRT').Visible = 'on';
      | else
      |     maskObj.getDialogControl('Container_LVRT').Visible = 'off';
      | end
      | 
      | % Note that the value of the bias is not handled here.
      | % See the Initialization tab
      mask DialogControl DescTextVar Prompt: -------------------------------------Three-phase VSC model---------------------------------------
      mask DialogControl Tab1 Prompt: Electrical parameters
      mask DialogControl Tab2 Prompt: Control parameters
      mask DialogControl Tab3 Prompt: Other parameters
      mask DialogControl Container_LVRT Prompt: LVRT
      mask DialogControl Tab4 Prompt: Power flow
      mask Display:
      | choice = get_param(gcb,'vscmod');
      | if strcmp(choice,'Phasor Quasi-EMT')
      |     disp('VSC\n\n')
      |     disp('\n\nPhasor\n\n')
      |     disp('\n\nQuasi-EMT')
      | elseif strcmp(choice,'EMT Average')
      |     disp('VSC\n')
      |     disp('\nEMT AVG')
      | elseif strcmp(choice,'EMT Switching')
      |     disp('VSC\n')
      |     disp('\nEMT SW')
      | elseif strcmp(choice,'Phasor I-1st')
      |     disp('VSC\n\n')
      |     disp('\n\nPhasor\n\n')
      |     disp('\n\nI 1st')
      | elseif strcmp(choice,'Phasor I-ref')
      |     disp('VSC\n\n')
      |     disp('\n\nPhasor\n\n')
      |     disp('\n\nI ref')
      | elseif strcmp(choice,'Phasor PQ-1st')
      |     disp('VSC\n\n')
      |     disp('\n\nPhasor\n\n')
      |     disp('\n\nPQ 1st')
      | end
  A1 : PMIOPort  Side=Right
  B1 : PMIOPort  Port=2  Side=Right
  C1 : PMIOPort  Port=3  Side=Right
  A2 : PMIOPort  Port=4  Side=Left
  B2 : PMIOPort  Port=5  Side=Left
  C2 : PMIOPort  Port=6  Side=Left
  tag scope: fg4=global, fg7=global
  wires:
  Constant/1 -> VSC1/1(Pset)
  [Pac7] -> Gain1/1
  Divide/1 -> [idc1]
  VSC1/1(m) -> Bus Selector2/1
  Constant2/1 -> VSC2/1(Qset)
  Bus Selector1/2 -> [Qac4]  "<Qabc>"
  Bus Selector1/1 -> [Pac4]  "<Pabc>"
  VSC2/1(m) -> Bus Selector1/1
  [vdc2] -> VSC2/2(Edc)
  [idc1] -> Unit Delay/1
  Unit Delay/1 -> DC-link/1(idc1)
  Unit Delay1/1 -> DC-link/2(idc2)
  [idc2] -> Unit Delay1/1
  Divide1/1 -> [idc2]
  DC-link/1(vdc1) -> [vdc1]
  DC-link/2(vdc2) -> [vdc2]
  Bus Selector2/2 -> [Qac7]  "<Qabc>"
  Bus Selector2/1 -> [Pac7]  "<Pabc>"
  Bus Selector2/3 -> [fg7]  "<f>"
  Bus Selector1/3 -> [fg4]  "<f>"
  Constant1/1 -> VSC1/2(Qset)
  Gain1/1 -> Divide/1
  [Pac4] -> Gain2/1
  Gain2/1 -> Divide1/1
  [vdc1] -> Saturation/1
  Saturation/1 -> Divide/2
  Saturation1/1 -> Divide1/2
  [vdc2] -> Saturation1/1
  connections:
  VSC1/LConn2 -- B1/RConn1
  VSC1/LConn3 -- C1/RConn1
  VSC2/LConn1 -- A2/RConn1
  VSC2/LConn2 -- B2/RConn1
  VSC2/LConn3 -- C2/RConn1
  VSC1/LConn1 -- A1/RConn1
